simulink model "euler321_I2B_12B_with_contracts_ALL_PP"  (R2017b)
settings: Solver=FixedStepDiscrete  StartTime=0.0  StopTime=10.0  FixedStep=0.010000  RelTol=1e-3  EnableMultiTasking=on
model workspace (MAT data in the model file):
  ContractValidatorBlocksMap = containers.Map
  ContractValidatorBlocksMap.serialization.keys = {'euler321_I2B_12B_with_contracts/euler321_I2B_12B_euler321_Spec/validator', 'euler321_I2B_12B_with_contracts_ALL/euler321_I2B_12B_euler321_Spec/validator'}
  ContractValidatorBlocksMap.serialization.values{1}.block = 'euler321_I2B_12B_with_contracts/euler321_I2B_12B_euler321_Spec/validator'
  ContractValidatorBlocksMap.serialization.values{1}.assumePorts = 0
  ContractValidatorBlocksMap.serialization.values{1}.guaranteePorts = 20
  ContractValidatorBlocksMap.serialization.values{1}.modeBlocksPorts = 0
  ContractValidatorBlocksMap.serialization.values{1}.portHandles.Inport = [576.090576172 577.090576172 578.090576172 579.090576172 580.090576172 581.090576172 582.090576172 583.090576172 584.090576172 585.090576172 586.090576172 587.090576172 588.090576172 589.090576172 590.090576172 591.090576172 592.090576172 593.090576172 594.090576172 595.090576172]
  ContractValidatorBlocksMap.serialization.values{1}.portHandles.Outport = 596.090576172
  ContractValidatorBlocksMap.serialization.values{1}.portHandles.Enable = []
  ContractValidatorBlocksMap.serialization.values{1}.portHandles.Trigger = []
  ContractValidatorBlocksMap.serialization.values{1}.portHandles.State = []
  ContractValidatorBlocksMap.serialization.values{1}.portHandles.LConn = []
  ContractValidatorBlocksMap.serialization.values{1}.portHandles.RConn = []
  ContractValidatorBlocksMap.serialization.values{1}.portHandles.Ifaction = []
  ContractValidatorBlocksMap.serialization.values{1}.portHandles.Reset = []
  ContractValidatorBlocksMap.serialization.values{1}.portConnectivity(1).Type = '1'
  ContractValidatorBlocksMap.serialization.values{1}.portConnectivity(1).Position = [6680 -1090]
  ContractValidatorBlocksMap.serialization.values{1}.portConnectivity(1).SrcBlock = 1677.00183105
  ContractValidatorBlocksMap.serialization.values{1}.portConnectivity(1).SrcPort = 0
  ContractValidatorBlocksMap.serialization.values{1}.portConnectivity(1).DstBlock = []
  ContractValidatorBlocksMap.serialization.values{1}.portConnectivity(1).DstPort = []
  ContractValidatorBlocksMap.serialization.values{1}.portConnectivity(2).Type = '2'
  ContractValidatorBlocksMap.serialization.values{1}.portConnectivity(2).Position = [6680 -1025]
  ContractValidatorBlocksMap.serialization.values{1}.portConnectivity(2).SrcBlock = 1681.00183105
  ContractValidatorBlocksMap.serialization.values{1}.portConnectivity(2).SrcPort = 0
  ContractValidatorBlocksMap.serialization.values{1}.portConnectivity(2).DstBlock = []
  ContractValidatorBlocksMap.serialization.values{1}.portConnectivity(2).DstPort = []
  ContractValidatorBlocksMap.serialization.values{1}.portConnectivity(3).Type = '3'
  ContractValidatorBlocksMap.serialization.values{1}.portConnectivity(3).Position = [6680 -960]
  ContractValidatorBlocksMap.serialization.values{1}.portConnectivity(3).SrcBlock = 1685.00170898
  ContractValidatorBlocksMap.serialization.values{1}.portConnectivity(3).SrcPort = 0
  ContractValidatorBlocksMap.serialization.values{1}.portConnectivity(3).DstBlock = []
  ContractValidatorBlocksMap.serialization.values{1}.portConnectivity(3).DstPort = []
  ContractValidatorBlocksMap.serialization.values{1}.portConnectivity(4).Type = '4'
  ContractValidatorBlocksMap.serialization.values{1}.portConnectivity(4).Position = [6680 -895]
  ContractValidatorBlocksMap.serialization.values{1}.portConnectivity(4).SrcBlock = 1689.00183105
  ContractValidatorBlocksMap.serialization.values{1}.portConnectivity(4).SrcPort = 0
  ContractValidatorBlocksMap.serialization.values{1}.portConnectivity(4).DstBlock = []
  ContractValidatorBlocksMap.serialization.values{1}.portConnectivity(4).DstPort = []
  ContractValidatorBlocksMap.serialization.values{1}.portConnectivity(5).Type = '5'
  ContractValidatorBlocksMap.serialization.values{1}.portConnectivity(5).Position = [6680 -830]
  ContractValidatorBlocksMap.serialization.values{1}.portConnectivity(5).SrcBlock = 1693.00146484
  ContractValidatorBlocksMap.serialization.values{1}.portConnectivity(5).SrcPort = 0
  ContractValidatorBlocksMap.serialization.values{1}.portConnectivity(5).DstBlock = []
  ContractValidatorBlocksMap.serialization.values{1}.portConnectivity(5).DstPort = []
  ContractValidatorBlocksMap.serialization.values{1}.portConnectivity(6).Type = '6'
  ContractValidatorBlocksMap.serialization.values{1}.portConnectivity(6).Position = [6680 -765]
  ContractValidatorBlocksMap.serialization.values{1}.portConnectivity(6).SrcBlock = 1697.00146484
  ContractValidatorBlocksMap.serialization.values{1}.portConnectivity(6).SrcPort = 0
  ContractValidatorBlocksMap.serialization.values{1}.portConnectivity(6).DstBlock = []
  ContractValidatorBlocksMap.serialization.values{1}.portConnectivity(6).DstPort = []
  ContractValidatorBlocksMap.serialization.values{1}.portConnectivity(7).Type = '7'
  ContractValidatorBlocksMap.serialization.values{1}.portConnectivity(7).Position = [6680 -700]
  ContractValidatorBlocksMap.serialization.values{1}.portConnectivity(7).SrcBlock = 1701.00183105
  ContractValidatorBlocksMap.serialization.values{1}.portConnectivity(7).SrcPort = 0
  ContractValidatorBlocksMap.serialization.values{1}.portConnectivity(7).DstBlock = []
  ContractValidatorBlocksMap.serialization.values{1}.portConnectivity(7).DstPort = []
  ContractValidatorBlocksMap.serialization.values{1}.portConnectivity(8).Type = '8'
  ContractValidatorBlocksMap.serialization.values{1}.portConnectivity(8).Position = [6680 -635]
  ContractValidatorBlocksMap.serialization.values{1}.portConnectivity(8).SrcBlock = 1705.00183105
  ContractValidatorBlocksMap.serialization.values{1}.portConnectivity(8).SrcPort = 0
  ContractValidatorBlocksMap.serialization.values{1}.portConnectivity(8).DstBlock = []
  ContractValidatorBlocksMap.serialization.values{1}.portConnectivity(8).DstPort = []
  ContractValidatorBlocksMap.serialization.values{1}.portConnectivity(9).Type = '9'
  ContractValidatorBlocksMap.serialization.values{1}.portConnectivity(9).Position = [6680 -570]
  ContractValidatorBlocksMap.serialization.values{1}.portConnectivity(9).SrcBlock = 1709.00134277
  ContractValidatorBlocksMap.serialization.values{1}.portConnectivity(9).SrcPort = 0
  ContractValidatorBlocksMap.serialization.values{1}.portConnectivity(9).DstBlock = []
  ContractValidatorBlocksMap.serialization.values{1}.portConnectivity(9).DstPort = []
  ContractValidatorBlocksMap.serialization.values{1}.portConnectivity(10).Type = '10'
  ContractValidatorBlocksMap.serialization.values{1}.portConnectivity(10).Position = [6680 -505]
  ContractValidatorBlocksMap.serialization.values{1}.portConnectivity(10).SrcBlock = 1713.00170898
  ContractValidatorBlocksMap.serialization.values{1}.portConnectivity(10).SrcPort = 0
  ContractValidatorBlocksMap.serialization.values{1}.portConnectivity(10).DstBlock = []
  ContractValidatorBlocksMap.serialization.values{1}.portConnectivity(10).DstPort = []
  ContractValidatorBlocksMap.serialization.values{1}.portConnectivity(11).Type = '11'
  ContractValidatorBlocksMap.serialization.values{1}.portConnectivity(11).Position = [6680 -440]
  ContractValidatorBlocksMap.serialization.values{1}.portConnectivity(11).SrcBlock = 1717.00183105
  ContractValidatorBlocksMap.serialization.values{1}.portConnectivity(11).SrcPort = 0
  ContractValidatorBlocksMap.serialization.values{1}.portConnectivity(11).DstBlock = []
  ContractValidatorBlocksMap.serialization.values{1}.portConnectivity(11).DstPort = []
  ContractValidatorBlocksMap.serialization.values{1}.portConnectivity(12).Type = '12'
  ContractValidatorBlocksMap.serialization.values{1}.portConnectivity(12).Position = [6680 -375]
  ContractValidatorBlocksMap.serialization.values{1}.portConnectivity(12).SrcBlock = 1721.00146484
  ContractValidatorBlocksMap.serialization.values{1}.portConnectivity(12).SrcPort = 0
  ContractValidatorBlocksMap.serialization.values{1}.portConnectivity(12).DstBlock = []
  ContractValidatorBlocksMap.serialization.values{1}.portConnectivity(12).DstPort = []
  ContractValidatorBlocksMap.serialization.values{1}.portConnectivity(13).Type = '13'
  ContractValidatorBlocksMap.serialization.values{1}.portConnectivity(13).Position = [6680 -310]
  ContractValidatorBlocksMap.serialization.values{1}.portConnectivity(13).SrcBlock = 1725.00170898
  ContractValidatorBlocksMap.serialization.values{1}.portConnectivity(13).SrcPort = 0
  ContractValidatorBlocksMap.serialization.values{1}.portConnectivity(13).DstBlock = []
  ContractValidatorBlocksMap.serialization.values{1}.portConnectivity(13).DstPort = []
  ContractValidatorBlocksMap.serialization.values{1}.portConnectivity(14).Type = '14'
  ContractValidatorBlocksMap.serialization.values{1}.portConnectivity(14).Position = [6680 -245]
  ContractValidatorBlocksMap.serialization.values{1}.portConnectivity(14).SrcBlock = 1729.00146484
  ContractValidatorBlocksMap.serialization.values{1}.portConnectivity(14).SrcPort = 0
  ContractValidatorBlocksMap.serialization.values{1}.portConnectivity(14).DstBlock = []
  ContractValidatorBlocksMap.serialization.values{1}.portConnectivity(14).DstPort = []
  ContractValidatorBlocksMap.serialization.values{1}.portConnectivity(15).Type = '15'
  ContractValidatorBlocksMap.serialization.values{1}.portConnectivity(15).Position = [6680 -180]
  ContractValidatorBlocksMap.serialization.values{1}.portConnectivity(15).SrcBlock = 1733.00183105
  ContractValidatorBlocksMap.serialization.values{1}.portConnectivity(15).SrcPort = 0
  ContractValidatorBlocksMap.serialization.values{1}.portConnectivity(15).DstBlock = []
  ContractValidatorBlocksMap.serialization.values{1}.portConnectivity(15).DstPort = []
  ContractValidatorBlocksMap.serialization.values{1}.portConnectivity(16).Type = '16'
  ContractValidatorBlocksMap.serialization.values{1}.portConnectivity(16).Position = [6680 -115]
  ContractValidatorBlocksMap.serialization.values{1}.portConnectivity(16).SrcBlock = 1737.00134277
  ContractValidatorBlocksMap.serialization.values{1}.portConnectivity(16).SrcPort = 0
  ContractValidatorBlocksMap.serialization.values{1}.portConnectivity(16).DstBlock = []
  ContractValidatorBlocksMap.serialization.values{1}.portConnectivity(16).DstPort = []
  ContractValidatorBlocksMap.serialization.values{1}.portConnectivity(17).Type = '17'
  ContractValidatorBlocksMap.serialization.values{1}.portConnectivity(17).Position = [6680 -50]
  ContractValidatorBlocksMap.serialization.values{1}.portConnectivity(17).SrcBlock = 1741.00146484
  ContractValidatorBlocksMap.serialization.values{1}.portConnectivity(17).SrcPort = 0
  ContractValidatorBlocksMap.serialization.values{1}.portConnectivity(17).DstBlock = []
  ContractValidatorBlocksMap.serialization.values{1}.portConnectivity(17).DstPort = []
  ContractValidatorBlocksMap.serialization.values{1}.portConnectivity(18).Type = '18'
  ContractValidatorBlocksMap.serialization.values{1}.portConnectivity(18).Position = [6680 15]
  ContractValidatorBlocksMap.serialization.values{1}.portConnectivity(18).SrcBlock = 1745.00183105
  ContractValidatorBlocksMap.serialization.values{1}.portConnectivity(18).SrcPort = 0
  ContractValidatorBlocksMap.serialization.values{1}.portConnectivity(18).DstBlock = []
  ContractValidatorBlocksMap.serialization.values{1}.portConnectivity(18).DstPort = []
  ContractValidatorBlocksMap.serialization.values{1}.portConnectivity(19).Type = '19'
  ContractValidatorBlocksMap.serialization.values{1}.portConnectivity(19).Position = [6680 80]
  ContractValidatorBlocksMap.serialization.values{1}.portConnectivity(19).SrcBlock = 1834.0020752
  ContractValidatorBlocksMap.serialization.values{1}.portConnectivity(19).SrcPort = 0
  ContractValidatorBlocksMap.serialization.values{1}.portConnectivity(19).DstBlock = []
  ContractValidatorBlocksMap.serialization.values{1}.portConnectivity(19).DstPort = []
  ContractValidatorBlocksMap.serialization.values{1}.portConnectivity(20).Type = '20'
  ContractValidatorBlocksMap.serialization.values{1}.portConnectivity(20).Position = [6680 145]
  ContractValidatorBlocksMap.serialization.values{1}.portConnectivity(20).SrcBlock = 1838.00195312
  ContractValidatorBlocksMap.serialization.values{1}.portConnectivity(20).SrcPort = 0
  ContractValidatorBlocksMap.serialization.values{1}.portConnectivity(20).DstBlock = []
  ContractValidatorBlocksMap.serialization.values{1}.portConnectivity(20).DstPort = []
  ContractValidatorBlocksMap.serialization.values{1}.portConnectivity(21).Type = '1'
  ContractValidatorBlocksMap.serialization.values{1}.portConnectivity(21).Position = [6855 -470]
  ContractValidatorBlocksMap.serialization.values{1}.portConnectivity(21).SrcBlock = []
  ContractValidatorBlocksMap.serialization.values{1}.portConnectivity(21).SrcPort = []
  ContractValidatorBlocksMap.serialization.values{1}.portConnectivity(21).DstBlock = 2655.00268555
  ContractValidatorBlocksMap.serialization.values{1}.portConnectivity(21).DstPort = 0
  ContractValidatorBlocksMap.serialization.values{2}.block = 'euler321_I2B_12B_with_contracts_ALL/euler321_I2B_12B_euler321_Spec/validator'
  ContractValidatorBlocksMap.serialization.values{2}.assumePorts = 0
  ContractValidatorBlocksMap.serialization.values{2}.guaranteePorts = 20
  ContractValidatorBlocksMap.serialization.values{2}.modeBlocksPorts = 0
  ContractValidatorBlocksMap.serialization.values{2}.portHandles.Inport = [10350.0007324 10351.0007324 10352.0007324 10353.0007324 10354.0007324 10355.0007324 10356.0007324 10357.0007324 10358.0007324 10359.0007324 10360.0007324 10361.0007324 10362.0007324 10363.0007324 10364.0007324 10365.0007324 10366.0007324 10367.0007324 10368.0007324 10369.0007324]
  ContractValidatorBlocksMap.serialization.values{2}.portHandles.Outport = 10370.0007324
  ContractValidatorBlocksMap.serialization.values{2}.portHandles.Enable = []
  ContractValidatorBlocksMap.serialization.values{2}.portHandles.Trigger = []
  ContractValidatorBlocksMap.serialization.values{2}.portHandles.State = []
  ContractValidatorBlocksMap.serialization.values{2}.portHandles.LConn = []
  ContractValidatorBlocksMap.serialization.values{2}.portHandles.RConn = []
  ContractValidatorBlocksMap.serialization.values{2}.portHandles.Ifaction = []
  ContractValidatorBlocksMap.serialization.values{2}.portHandles.Reset = []
  ContractValidatorBlocksMap.serialization.values{2}.portConnectivity(1).Type = '1'
  ContractValidatorBlocksMap.serialization.values{2}.portConnectivity(1).Position = [6680 -1090]
  ContractValidatorBlocksMap.serialization.values{2}.portConnectivity(1).SrcBlock = 9376.00109863
  ContractValidatorBlocksMap.serialization.values{2}.portConnectivity(1).SrcPort = 0
  ContractValidatorBlocksMap.serialization.values{2}.portConnectivity(1).DstBlock = []
  ContractValidatorBlocksMap.serialization.values{2}.portConnectivity(1).DstPort = []
  ContractValidatorBlocksMap.serialization.values{2}.portConnectivity(2).Type = '2'
  ContractValidatorBlocksMap.serialization.values{2}.portConnectivity(2).Position = [6680 -1025]
  ContractValidatorBlocksMap.serialization.values{2}.portConnectivity(2).SrcBlock = 9380.00109863
  ContractValidatorBlocksMap.serialization.values{2}.portConnectivity(2).SrcPort = 0
  ContractValidatorBlocksMap.serialization.values{2}.portConnectivity(2).DstBlock = []
  ContractValidatorBlocksMap.serialization.values{2}.portConnectivity(2).DstPort = []
  ContractValidatorBlocksMap.serialization.values{2}.portConnectivity(3).Type = '3'
  ContractValidatorBlocksMap.serialization.values{2}.portConnectivity(3).Position = [6680 -960]
  ContractValidatorBlocksMap.serialization.values{2}.portConnectivity(3).SrcBlock = 9384.00109863
  ContractValidatorBlocksMap.serialization.values{2}.portConnectivity(3).SrcPort = 0
  ContractValidatorBlocksMap.serialization.values{2}.portConnectivity(3).DstBlock = []
  ContractValidatorBlocksMap.serialization.values{2}.portConnectivity(3).DstPort = []
  ContractValidatorBlocksMap.serialization.values{2}.portConnectivity(4).Type = '4'
  ContractValidatorBlocksMap.serialization.values{2}.portConnectivity(4).Position = [6680 -895]
  ContractValidatorBlocksMap.serialization.values{2}.portConnectivity(4).SrcBlock = 9388.00109863
  ContractValidatorBlocksMap.serialization.values{2}.portConnectivity(4).SrcPort = 0
  ContractValidatorBlocksMap.serialization.values{2}.portConnectivity(4).DstBlock = []
  ContractValidatorBlocksMap.serialization.values{2}.portConnectivity(4).DstPort = []
  ContractValidatorBlocksMap.serialization.values{2}.portConnectivity(5).Type = '5'
  ContractValidatorBlocksMap.serialization.values{2}.portConnectivity(5).Position = [6680 -830]
  ContractValidatorBlocksMap.serialization.values{2}.portConnectivity(5).SrcBlock = 9392.00109863
  ContractValidatorBlocksMap.serialization.values{2}.portConnectivity(5).SrcPort = 0
  ContractValidatorBlocksMap.serialization.values{2}.portConnectivity(5).DstBlock = []
  ContractValidatorBlocksMap.serialization.values{2}.portConnectivity(5).DstPort = []
  ContractValidatorBlocksMap.serialization.values{2}.portConnectivity(6).Type = '6'
  ContractValidatorBlocksMap.serialization.values{2}.portConnectivity(6).Position = [6680 -765]
  ContractValidatorBlocksMap.serialization.values{2}.portConnectivity(6).SrcBlock = 9396.00109863
  ContractValidatorBlocksMap.serialization.values{2}.portConnectivity(6).SrcPort = 0
  ContractValidatorBlocksMap.serialization.values{2}.portConnectivity(6).DstBlock = []
  ContractValidatorBlocksMap.serialization.values{2}.portConnectivity(6).DstPort = []
  ContractValidatorBlocksMap.serialization.values{2}.portConnectivity(7).Type = '7'
  ContractValidatorBlocksMap.serialization.values{2}.portConnectivity(7).Position = [6680 -700]
  ContractValidatorBlocksMap.serialization.values{2}.portConnectivity(7).SrcBlock = 9400.00109863
  ContractValidatorBlocksMap.serialization.values{2}.portConnectivity(7).SrcPort = 0
  ContractValidatorBlocksMap.serialization.values{2}.portConnectivity(7).DstBlock = []
  ContractValidatorBlocksMap.serialization.values{2}.portConnectivity(7).DstPort = []
  ContractValidatorBlocksMap.serialization.values{2}.portConnectivity(8).Type = '8'
  ContractValidatorBlocksMap.serialization.values{2}.portConnectivity(8).Position = [6680 -635]
  ContractValidatorBlocksMap.serialization.values{2}.portConnectivity(8).SrcBlock = 9404.00109863
  ContractValidatorBlocksMap.serialization.values{2}.portConnectivity(8).SrcPort = 0
  ContractValidatorBlocksMap.serialization.values{2}.portConnectivity(8).DstBlock = []
  ContractValidatorBlocksMap.serialization.values{2}.portConnectivity(8).DstPort = []
  ContractValidatorBlocksMap.serialization.values{2}.portConnectivity(9).Type = '9'
  ContractValidatorBlocksMap.serialization.values{2}.portConnectivity(9).Position = [6680 -570]
  ContractValidatorBlocksMap.serialization.values{2}.portConnectivity(9).SrcBlock = 9408.00109863
  ContractValidatorBlocksMap.serialization.values{2}.portConnectivity(9).SrcPort = 0
  ContractValidatorBlocksMap.serialization.values{2}.portConnectivity(9).DstBlock = []
  ContractValidatorBlocksMap.serialization.values{2}.portConnectivity(9).DstPort = []
  ContractValidatorBlocksMap.serialization.values{2}.portConnectivity(10).Type = '10'
  ContractValidatorBlocksMap.serialization.values{2}.portConnectivity(10).Position = [6680 -505]
  ContractValidatorBlocksMap.serialization.values{2}.portConnectivity(10).SrcBlock = 9412.00109863
  ContractValidatorBlocksMap.serialization.values{2}.portConnectivity(10).SrcPort = 0
  ContractValidatorBlocksMap.serialization.values{2}.portConnectivity(10).DstBlock = []
  ContractValidatorBlocksMap.serialization.values{2}.portConnectivity(10).DstPort = []
  ContractValidatorBlocksMap.serialization.values{2}.portConnectivity(11).Type = '11'
  ContractValidatorBlocksMap.serialization.values{2}.portConnectivity(11).Position = [6680 -440]
  ContractValidatorBlocksMap.serialization.values{2}.portConnectivity(11).SrcBlock = 9416.00109863
  ContractValidatorBlocksMap.serialization.values{2}.portConnectivity(11).SrcPort = 0
  ContractValidatorBlocksMap.serialization.values{2}.portConnectivity(11).DstBlock = []
  ContractValidatorBlocksMap.serialization.values{2}.portConnectivity(11).DstPort = []
  ContractValidatorBlocksMap.serialization.values{2}.portConnectivity(12).Type = '12'
  ContractValidatorBlocksMap.serialization.values{2}.portConnectivity(12).Position = [6680 -375]
  ContractValidatorBlocksMap.serialization.values{2}.portConnectivity(12).SrcBlock = 9420.00109863
  ContractValidatorBlocksMap.serialization.values{2}.portConnectivity(12).SrcPort = 0
  ContractValidatorBlocksMap.serialization.values{2}.portConnectivity(12).DstBlock = []
  ContractValidatorBlocksMap.serialization.values{2}.portConnectivity(12).DstPort = []
  ContractValidatorBlocksMap.serialization.values{2}.portConnectivity(13).Type = '13'
  ContractValidatorBlocksMap.serialization.values{2}.portConnectivity(13).Position = [6680 -310]
  ContractValidatorBlocksMap.serialization.values{2}.portConnectivity(13).SrcBlock = 9424.00109863
  ContractValidatorBlocksMap.serialization.values{2}.portConnectivity(13).SrcPort = 0
  ContractValidatorBlocksMap.serialization.values{2}.portConnectivity(13).DstBlock = []
  ContractValidatorBlocksMap.serialization.values{2}.portConnectivity(13).DstPort = []
  ContractValidatorBlocksMap.serialization.values{2}.portConnectivity(14).Type = '14'
  ContractValidatorBlocksMap.serialization.values{2}.portConnectivity(14).Position = [6680 -245]
  ContractValidatorBlocksMap.serialization.values{2}.portConnectivity(14).SrcBlock = 9428.00109863
  ContractValidatorBlocksMap.serialization.values{2}.portConnectivity(14).SrcPort = 0
  ContractValidatorBlocksMap.serialization.values{2}.portConnectivity(14).DstBlock = []
  ContractValidatorBlocksMap.serialization.values{2}.portConnectivity(14).DstPort = []
  ContractValidatorBlocksMap.serialization.values{2}.portConnectivity(15).Type = '15'
  ContractValidatorBlocksMap.serialization.values{2}.portConnectivity(15).Position = [6680 -180]
  ContractValidatorBlocksMap.serialization.values{2}.portConnectivity(15).SrcBlock = 9432.00109863
  ContractValidatorBlocksMap.serialization.values{2}.portConnectivity(15).SrcPort = 0
  ContractValidatorBlocksMap.serialization.values{2}.portConnectivity(15).DstBlock = []
  ContractValidatorBlocksMap.serialization.values{2}.portConnectivity(15).DstPort = []
  ContractValidatorBlocksMap.serialization.values{2}.portConnectivity(16).Type = '16'
  ContractValidatorBlocksMap.serialization.values{2}.portConnectivity(16).Position = [6680 -115]
  ContractValidatorBlocksMap.serialization.values{2}.portConnectivity(16).SrcBlock = 9436.00109863
  ContractValidatorBlocksMap.serialization.values{2}.portConnectivity(16).SrcPort = 0
  ContractValidatorBlocksMap.serialization.values{2}.portConnectivity(16).DstBlock = []
  ContractValidatorBlocksMap.serialization.values{2}.portConnectivity(16).DstPort = []
  ContractValidatorBlocksMap.serialization.values{2}.portConnectivity(17).Type = '17'
  ContractValidatorBlocksMap.serialization.values{2}.portConnectivity(17).Position = [6680 -50]
  ContractValidatorBlocksMap.serialization.values{2}.portConnectivity(17).SrcBlock = 9440.00109863
  ContractValidatorBlocksMap.serialization.values{2}.portConnectivity(17).SrcPort = 0
  ContractValidatorBlocksMap.serialization.values{2}.portConnectivity(17).DstBlock = []
  ContractValidatorBlocksMap.serialization.values{2}.portConnectivity(17).DstPort = []
  ContractValidatorBlocksMap.serialization.values{2}.portConnectivity(18).Type = '18'
  ContractValidatorBlocksMap.serialization.values{2}.portConnectivity(18).Position = [6680 15]
  ContractValidatorBlocksMap.serialization.values{2}.portConnectivity(18).SrcBlock = 9444.00109863
  ContractValidatorBlocksMap.serialization.values{2}.portConnectivity(18).SrcPort = 0
  ContractValidatorBlocksMap.serialization.values{2}.portConnectivity(18).DstBlock = []
  ContractValidatorBlocksMap.serialization.values{2}.portConnectivity(18).DstPort = []
  ContractValidatorBlocksMap.serialization.values{2}.portConnectivity(19).Type = '19'
  ContractValidatorBlocksMap.serialization.values{2}.portConnectivity(19).Position = [6680 80]
  ContractValidatorBlocksMap.serialization.values{2}.portConnectivity(19).SrcBlock = 9448.00109863
  ContractValidatorBlocksMap.serialization.values{2}.portConnectivity(19).SrcPort = 0
  ContractValidatorBlocksMap.serialization.values{2}.portConnectivity(19).DstBlock = []
  ContractValidatorBlocksMap.serialization.values{2}.portConnectivity(19).DstPort = []
  ContractValidatorBlocksMap.serialization.values{2}.portConnectivity(20).Type = '20'
  ContractValidatorBlocksMap.serialization.values{2}.portConnectivity(20).Position = [6680 145]
  ContractValidatorBlocksMap.serialization.values{2}.portConnectivity(20).SrcBlock = 9452.00109863
  ContractValidatorBlocksMap.serialization.values{2}.portConnectivity(20).SrcPort = 0
  ContractValidatorBlocksMap.serialization.values{2}.portConnectivity(20).DstBlock = []
  ContractValidatorBlocksMap.serialization.values{2}.portConnectivity(20).DstPort = []
  ContractValidatorBlocksMap.serialization.values{2}.portConnectivity(21).Type = '1'
  ContractValidatorBlocksMap.serialization.values{2}.portConnectivity(21).Position = [6855 -470]
  ContractValidatorBlocksMap.serialization.values{2}.portConnectivity(21).SrcBlock = []
  ContractValidatorBlocksMap.serialization.values{2}.portConnectivity(21).SrcPort = []
  ContractValidatorBlocksMap.serialization.values{2}.portConnectivity(21).DstBlock = 9756.01013184
  ContractValidatorBlocksMap.serialization.values{2}.portConnectivity(21).DstPort = 0
  ContractValidatorBlocksMap.serialization.uniformity = 0
  ContractValidatorBlocksMap.serialization.keyType = 'char'
  ContractValidatorBlocksMap.serialization.valueType = 'any'
  already_pp = 1
undefined symbols (not defined in the file): contractAfterSimulation, contractBeforeSimulation, ContractBlock, ContractGuaranteeBlock, ContractValidatorBlock, saveValidatorParameters
(part 1 of 2)
settings Model: Creator=elliocm  LastModifiedBy=hbourbou
settings DataIOCC: LimitDataPoints=on  SaveFormat=StructureWithTime  SignalLoggingSaveFormat=ModelDataLogs
settings OptimizationCC: ExpressionDepthLimit=2147483647  LifeSpan=inf
settings DebuggingCC: AlgebraicLoopMsg=error  ArtificialAlgebraicLoopMsg=error  UnderspecifiedInitializationDetection=Classic  MergeDetectMultiDrivingBlocksExec=none  SolverPrmCheckMsg=warning  SingleTaskRateTransMsg=error  FcnCallInpInsideContextMsg=warning  StateNameClashWarn=warning  SFUnexpectedBacktrackingDiag=warning  SFNoUnconditionalDefaultTransitionDiag=warning  SFExecutionAtInitializationDiag=none
settings HardwareCC: ProdBitPerPointer=32  ProdBitPerSizeT=32  ProdBitPerPtrDiffT=32  ProdLargestAtomicFloat=None  ProdIntDivRoundTo=Undefined  ProdEndianess=Unspecified  ProdWordSize=32  ProdHWDeviceType=32-bit Generic
settings ModelReferenceCC: PropagateSignalLabelsOutOfModel=off
settings CodeAppCC: StateflowObjectComments=on
settings GRTTargetCC: TargetLangStandard=C89/C90 (ANSI)  GeneratePreprocessorConditionals=Disable all  CombineOutputUpdateFcns=off  GRTInterface=on
settings ConfigComp: CovMetricSettings=dw  CovHtmlReporting=on  CovSaveCumulativeToWorkspaceVar=on  CovSaveSingleToWorkspaceVar=on  CovExternalEMLEnable=off

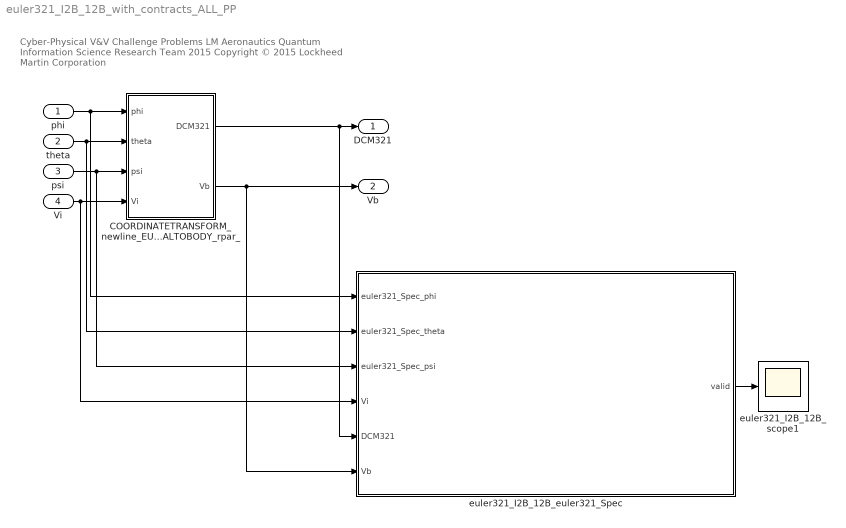
== system euler321_I2B_12B_with_contracts_ALL_PP ==
  note: Cyber-Physical V&V Challenge Problems
      | LM Aeronautics Quantum Information Science Research Team 2015
      | Copyright © 2015 Lockheed Martin Corporation
  phi : Inport  OutDataTypeStr=double
  theta : Inport  Port=2  OutDataTypeStr=double
  psi : Inport  Port=3  OutDataTypeStr=double
  Vi : Inport  Port=4  OutDataTypeStr=double  PortDimensions=3
  COORDINATETRANSFORM_newline_EULER321_newline__lpar_INERTIALTOBODY_rpar_ : Subsystem  TreatAsAtomicUnit=on
  euler321_I2B_12B_euler321_Spec : Subsystem  TreatAsAtomicUnit=on  mask(ContractBlock){ContractBlockType=ContractBlock}
      mask init:
      | set_param(gcb, 'LinkStatus', 'none');
      mask DialogControl DescTextVar Prompt: Contract block
      mask Display:
      | text(0.5, 0.5, '{\bf\fontsize{20}Contract}', 'hor', 'center', 'texmode','on');
      | blocks = find_system(gcb, 'LookUnderMasks','all', 'SearchDepth',1,'BlockType','Inport');
      | for i = 1 : length(blocks)
      |     blockName = get_param(blocks(i), 'Name');
      |     [path, blockName] = fileparts(char(blockName));
      |     port_label('input', i, blockName);
      | end
      | 
      | blocks = find_system(gcb, 'LookUnderMasks','all', 'SearchDepth',1,'BlockType','Outport');
      | for i = 1 : length(blocks)
      |     blockName = get_param(blocks(i), 'Name');
      |     [path, blockName] = fileparts(char(blockName));
      |     port_label('output', i, blockName);
      | end
  euler321_I2B_12B_scope1 : Scope
  DCM321 : Outport  VectorParamsAs1DForOutWhenUnconnected=off
  Vb : Outport  Port=2  VectorParamsAs1DForOutWhenUnconnected=off
  wires:
  COORDINATETRANSFORM_newline_EULER321_newline__lpar_INERTIALTOBODY_rpar_/1(DCM321) -> euler321_I2B_12B_euler321_Spec/5(DCM321), DCM321/1
  COORDINATETRANSFORM_newline_EULER321_newline__lpar_INERTIALTOBODY_rpar_/2(Vb) -> euler321_I2B_12B_euler321_Spec/6(Vb), Vb/1
  phi/1 -> euler321_I2B_12B_euler321_Spec/1(euler321_Spec_phi), COORDINATETRANSFORM_newline_EULER321_newline__lpar_INERTIALTOBODY_rpar_/1(phi)
  theta/1 -> euler321_I2B_12B_euler321_Spec/2(euler321_Spec_theta), COORDINATETRANSFORM_newline_EULER321_newline__lpar_INERTIALTOBODY_rpar_/2(theta)
  psi/1 -> euler321_I2B_12B_euler321_Spec/3(euler321_Spec_psi), COORDINATETRANSFORM_newline_EULER321_newline__lpar_INERTIALTOBODY_rpar_/3(psi)
  Vi/1 -> COORDINATETRANSFORM_newline_EULER321_newline__lpar_INERTIALTOBODY_rpar_/4(Vi), euler321_I2B_12B_euler321_Spec/4(Vi)
  euler321_I2B_12B_euler321_Spec/1(valid) -> euler321_I2B_12B_scope1/1

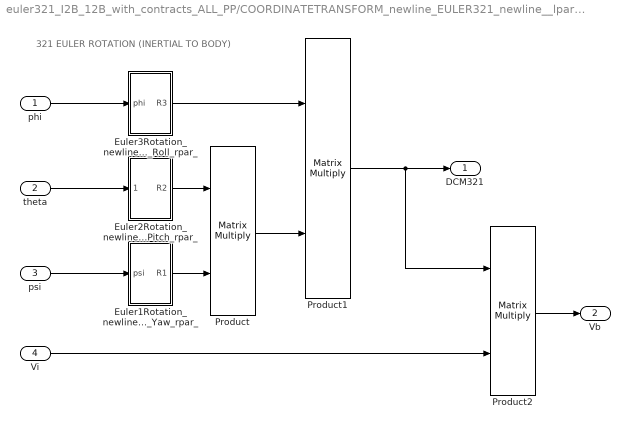
== system euler321_I2B_12B_with_contracts_ALL_PP/COORDINATETRANSFORM_newline_EULER321_newline__lpar_INERTIALTOBODY_rpar_ ==
  note: 321 EULER ROTATION (INERTIAL TO BODY)
  phi : Inport
  theta : Inport  Port=2
  psi : Inport  Port=3
  Vi : Inport  Port=4
  Euler1Rotation_newline__lpar_Yaw_rpar_ : Subsystem  TreatAsAtomicUnit=on
  Euler2Rotation_newline__lpar_Pitch_rpar_ : Subsystem  TreatAsAtomicUnit=on
  Euler3Rotation_newline__lpar_Roll_rpar_ : Subsystem  TreatAsAtomicUnit=on
  Product : Product  Multiplication=Matrix(*)  RndMeth=Zero
  Product1 : Product  Multiplication=Matrix(*)  RndMeth=Zero
  Product2 : Product  Multiplication=Matrix(*)  RndMeth=Zero
  DCM321 : Outport  VectorParamsAs1DForOutWhenUnconnected=off
  Vb : Outport  Port=2  VectorParamsAs1DForOutWhenUnconnected=off
  wires:
  Euler2Rotation_newline__lpar_Pitch_rpar_/1(R2) -> Product/1
  Euler1Rotation_newline__lpar_Yaw_rpar_/1(R1) -> Product/2
  Euler3Rotation_newline__lpar_Roll_rpar_/1(R3) -> Product1/1
  Product/1 -> Product1/2
  Product1/1 -> DCM321/1, Product2/1
  Product2/1 -> Vb/1
  phi/1 -> Euler3Rotation_newline__lpar_Roll_rpar_/1(phi)
  theta/1 -> Euler2Rotation_newline__lpar_Pitch_rpar_/1(theta)
  psi/1 -> Euler1Rotation_newline__lpar_Yaw_rpar_/1(psi)
  Vi/1 -> Product2/2

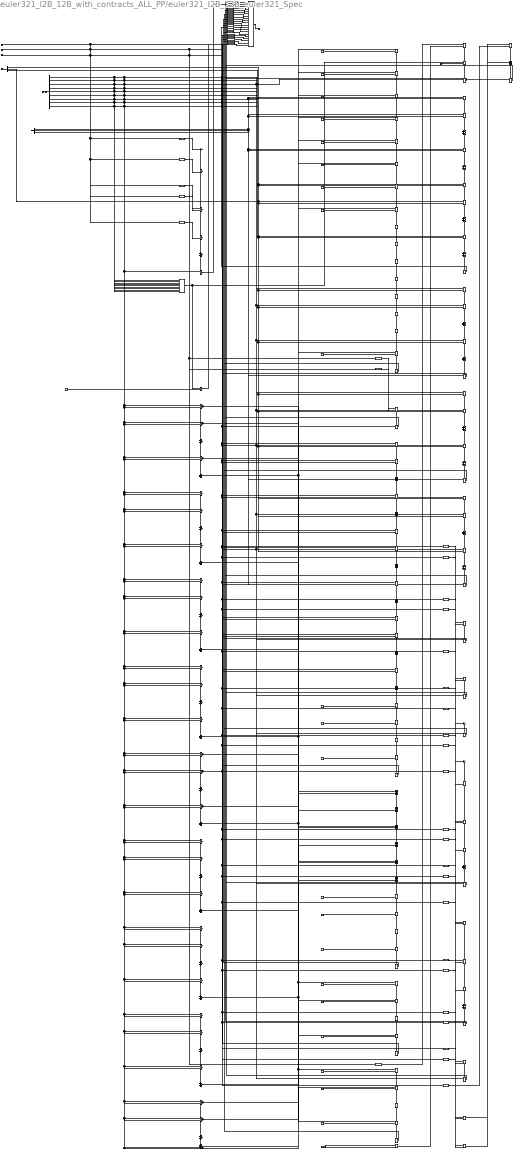
== system euler321_I2B_12B_with_contracts_ALL_PP/euler321_I2B_12B_euler321_Spec ==
  euler321_Spec_phi : Inport  OutDataTypeStr=double
  euler321_Spec_theta : Inport  Port=2  OutDataTypeStr=double
  euler321_Spec_psi : Inport  Port=3  OutDataTypeStr=double
  Vi : Inport  Port=4
  DCM321 : Inport  Port=5
  Vb : Inport  Port=6
  Demux : Demux  Outputs=3
  Demux1 : Demux  Outputs=3
  Demux3 : Demux  Outputs=9
  EUL_001_1 : Subsystem  TreatAsAtomicUnit=on  mask(ContractGuaranteeBlock){ContractBlockType=ContractGuaranteeBlock}
      mask init:
      | set_param(gcb, 'LinkStatus', 'none');
      mask DialogControl DescTextVar Prompt: Guarantee block
  EUL_001_2 : Subsystem  TreatAsAtomicUnit=on  mask(ContractGuaranteeBlock){ContractBlockType=ContractGuaranteeBlock}
      mask init:
      | set_param(gcb, 'LinkStatus', 'none');
      mask DialogControl DescTextVar Prompt: Guarantee block
  EUL_001_3 : Subsystem  TreatAsAtomicUnit=on  mask(ContractGuaranteeBlock){ContractBlockType=ContractGuaranteeBlock}
      mask init:
      | set_param(gcb, 'LinkStatus', 'none');
      mask DialogControl DescTextVar Prompt: Guarantee block
  EUL_001_4 : Subsystem  TreatAsAtomicUnit=on  mask(ContractGuaranteeBlock){ContractBlockType=ContractGuaranteeBlock}
      mask init:
      | set_param(gcb, 'LinkStatus', 'none');
      mask DialogControl DescTextVar Prompt: Guarantee block
  EUL_001_5 : Subsystem  TreatAsAtomicUnit=on  mask(ContractGuaranteeBlock){ContractBlockType=ContractGuaranteeBlock}
      mask init:
      | set_param(gcb, 'LinkStatus', 'none');
      mask DialogControl DescTextVar Prompt: Guarantee block
  EUL_001_6 : Subsystem  TreatAsAtomicUnit=on  mask(ContractGuaranteeBlock){ContractBlockType=ContractGuaranteeBlock}
      mask init:
      | set_param(gcb, 'LinkStatus', 'none');
      mask DialogControl DescTextVar Prompt: Guarantee block
  EUL_001_7 : Subsystem  TreatAsAtomicUnit=on  mask(ContractGuaranteeBlock){ContractBlockType=ContractGuaranteeBlock}
      mask init:
      | set_param(gcb, 'LinkStatus', 'none');
      mask DialogControl DescTextVar Prompt: Guarantee block
  EUL_001_8 : Subsystem  TreatAsAtomicUnit=on  mask(ContractGuaranteeBlock){ContractBlockType=ContractGuaranteeBlock}
      mask init:
      | set_param(gcb, 'LinkStatus', 'none');
      mask DialogControl DescTextVar Prompt: Guarantee block
  EUL_001_9 : Subsystem  TreatAsAtomicUnit=on  mask(ContractGuaranteeBlock){ContractBlockType=ContractGuaranteeBlock}
      mask init:
      | set_param(gcb, 'LinkStatus', 'none');
      mask DialogControl DescTextVar Prompt: Guarantee block
  EUL_002_1 : Subsystem  TreatAsAtomicUnit=on  mask(ContractGuaranteeBlock){ContractBlockType=ContractGuaranteeBlock}
      mask init:
      | set_param(gcb, 'LinkStatus', 'none');
      mask DialogControl DescTextVar Prompt: Guarantee block
  EUL_002_2 : Subsystem  TreatAsAtomicUnit=on  mask(ContractGuaranteeBlock){ContractBlockType=ContractGuaranteeBlock}
      mask init:
      | set_param(gcb, 'LinkStatus', 'none');
      mask DialogControl DescTextVar Prompt: Guarantee block
  EUL_002_3 : Subsystem  TreatAsAtomicUnit=on  mask(ContractGuaranteeBlock){ContractBlockType=ContractGuaranteeBlock}
      mask init:
      | set_param(gcb, 'LinkStatus', 'none');
      mask DialogControl DescTextVar Prompt: Guarantee block
  EUL_003 : Subsystem  TreatAsAtomicUnit=on  mask(ContractGuaranteeBlock){ContractBlockType=ContractGuaranteeBlock}
      mask init:
      | set_param(gcb, 'LinkStatus', 'none');
      mask DialogControl DescTextVar Prompt: Guarantee block
  EUL_004 : Subsystem  TreatAsAtomicUnit=on  mask(ContractGuaranteeBlock){ContractBlockType=ContractGuaranteeBlock}
      mask init:
      | set_param(gcb, 'LinkStatus', 'none');
      mask DialogControl DescTextVar Prompt: Guarantee block
  EUL_006_1 : Subsystem  TreatAsAtomicUnit=on  mask(ContractGuaranteeBlock){ContractBlockType=ContractGuaranteeBlock}
      mask init:
      | set_param(gcb, 'LinkStatus', 'none');
      mask DialogControl DescTextVar Prompt: Guarantee block
  EUL_006_2 : Subsystem  TreatAsAtomicUnit=on  mask(ContractGuaranteeBlock){ContractBlockType=ContractGuaranteeBlock}
      mask init:
      | set_param(gcb, 'LinkStatus', 'none');
      mask DialogControl DescTextVar Prompt: Guarantee block
  EUL_006_3 : Subsystem  TreatAsAtomicUnit=on  mask(ContractGuaranteeBlock){ContractBlockType=ContractGuaranteeBlock}
      mask init:
      | set_param(gcb, 'LinkStatus', 'none');
      mask DialogControl DescTextVar Prompt: Guarantee block
  EUL_006_4 : Subsystem  TreatAsAtomicUnit=on  mask(ContractGuaranteeBlock){ContractBlockType=ContractGuaranteeBlock}
      mask init:
      | set_param(gcb, 'LinkStatus', 'none');
      mask DialogControl DescTextVar Prompt: Guarantee block
  EUL_007 : Subsystem  TreatAsAtomicUnit=on  mask(ContractGuaranteeBlock){ContractBlockType=ContractGuaranteeBlock}
      mask init:
      | set_param(gcb, 'LinkStatus', 'none');
      mask DialogControl DescTextVar Prompt: Guarantee block
  EUL_008 : Subsystem  TreatAsAtomicUnit=on  mask(ContractGuaranteeBlock){ContractBlockType=ContractGuaranteeBlock}
      mask init:
      | set_param(gcb, 'LinkStatus', 'none');
      mask DialogControl DescTextVar Prompt: Guarantee block
  Reshape : Reshape
  abs_call : Subsystem  TreatAsAtomicUnit=on
  c1xc1Transpose_operator : Sum  OutDataTypeStr=double
  c1xc2Transpose_operator : Sum  OutDataTypeStr=double
  c1xc3Transpose_operator : Sum  OutDataTypeStr=double
  c2xc2Transpose_operator : Sum  OutDataTypeStr=double
  c2xc3Transpose_operator : Sum  OutDataTypeStr=double
  c3xc3Transpose_operator : Sum  OutDataTypeStr=double
  det_3x3_call : Subsystem  TreatAsAtomicUnit=on
  r1xr1Transpose_operator : Sum  OutDataTypeStr=double
  r1xr2Transpose_operator : Sum  OutDataTypeStr=double
  r1xr3Transpose_operator : Sum  OutDataTypeStr=double
  r2xr1Transpose_operator : Sum  OutDataTypeStr=double
  r2xr2Transpose_operator : Sum  OutDataTypeStr=double
  r2xr3Transpose_operator : Sum  OutDataTypeStr=double
  r3xr1Transpose_operator : Sum  OutDataTypeStr=double
  r3xr2Transpose_operator : Sum  OutDataTypeStr=double
  r3xr3Transpose_operator : Sum  OutDataTypeStr=double
  spec113_operator : RelationalOperator  Operator===  OutDataTypeStr=boolean  RndMeth=Simplest
  spec123_operator : RelationalOperator  Operator===  OutDataTypeStr=boolean  RndMeth=Simplest
  spec145_operator : RelationalOperator  Operator===  OutDataTypeStr=boolean  RndMeth=Simplest
  spec169_operator : RelationalOperator  Operator===  OutDataTypeStr=boolean  RndMeth=Simplest
  spec177_operator : RelationalOperator  Operator===  OutDataTypeStr=boolean  RndMeth=Simplest
  spec187_operator : RelationalOperator  Operator===  OutDataTypeStr=boolean  RndMeth=Simplest
  spec197_operator : RelationalOperator  Operator===  OutDataTypeStr=boolean  RndMeth=Simplest
  spec217_operator : RelationalOperator  Operator===  OutDataTypeStr=boolean  RndMeth=Simplest
  spec237_operator : RelationalOperator  Operator===  OutDataTypeStr=boolean  RndMeth=Simplest
  spec257_operator : RelationalOperator  Operator===  OutDataTypeStr=boolean  RndMeth=Simplest
  spec292_operator : RelationalOperator  Operator===  OutDataTypeStr=boolean  RndMeth=Simplest
  spec319_operator : Subsystem  TreatAsAtomicUnit=on
  spec432_operator : Logic  AllPortsSameDT=off  OutDataTypeStr=boolean
  spec449_operator : Logic  AllPortsSameDT=off  OutDataTypeStr=boolean
  spec466_operator : Logic  AllPortsSameDT=off  OutDataTypeStr=boolean
  spec483_operator : Logic  AllPortsSameDT=off  OutDataTypeStr=boolean
  spec67_operator : RelationalOperator  Operator===  OutDataTypeStr=boolean  RndMeth=Simplest
  spec689_operator : Logic  AllPortsSameDT=off  OutDataTypeStr=boolean
  spec694_operator : RelationalOperator  Operator===  OutDataTypeStr=boolean  RndMeth=Simplest
  spec694_rhs_2 : Constant  Value=1.0  OutDataTypeStr=double
  spec91_operator : RelationalOperator  Operator===  OutDataTypeStr=boolean  RndMeth=Simplest
  validator : M-S-Function  LoadFcn=saveValidatorParameters(gcb);  InitFcn=contractBeforeSimulation();  StopFcn=contractAfterSimulation();  FunctionName=contract  mask(ContractValidatorBlock){assumePorts=0, guaranteePorts=20, modePorts=0, ContractBlockType=ContractValidatorBlock, createInportsCheckbox=off}
      mask prompts: assumePorts "Assume ports     :"; guaranteePorts "Guarantee ports :"; modePorts "Mode ports        :"; createInportsCheckbox "Create inports and connect them automatically"
      mask init:
      | set_param(gcb,'LinkStatus','none');
      | contract_callback('inputs_callback',gcb);
      mask DialogControl DescTextVar Prompt: The validator block implements the following logic: <br> <br> <b>Sofar</b>(assume<sub>1</sub> <b>&#8743;</b> assume<sub>2</sub> <b>&#8743;</b> ... assume<sub>k</sub>) <b>&rarr;</b> (guarantee<sub>1</sub> <b>&#8743;</b> guarantee<sub>2</sub> <b>&#8743;</b> ... guarantee<sub>m</sub> <b>&#8743;</b>  mode<sub>1</sub> <b>&#8743;</b> mode<sub>2</sub> <b>&#8743;</b> ... <b>&#8743;</b> mode<sub>n</sub> )<br> where mode<sub>i</sub> = require<sub>i</sub> <b>&rarr;</b> ensure<sub>i</sub>
      mask Display:
      | color('black');
      | port_label('input',1,'guarantee');
      | port_label('input',2,'guarantee');
      | port_label('input',3,'guarantee');
      | port_label('input',4,'guarantee');
      | port_label('input',5,'guarantee');
      | port_label('input',6,'guarantee');
      | port_label('input',7,'guarantee');
      | port_label('input',8,'guarantee');
      | port_label('input',9,'guarantee');
      | port_label('input',10,'guarantee');
      | port_label('input',11,'guarantee');
      | port_label('input',12,'guarantee');
      | port_label('input',13,'guarantee');
      | port_label('input',14,'guarantee');
      | port_label('input',15,'guarantee');
      | port_label('input',16,'guarantee');
      | port_label('input',17,'guarantee');
      | port_label('input',18,'guarantee');
      | port_label('input',19,'guarantee');
      | port_label('input',20,'guarantee');
      | port_label('output',1,'valid');
  xxeuler321_Spec_100_operator : Sum  OutDataTypeStr=double
  xxeuler321_Spec_101_cos_call : Trigonometry  Operator=cos
  xxeuler321_Spec_102_sin_call : Trigonometry
  xxeuler321_Spec_103_sin_call : Trigonometry
  xxeuler321_Spec_104_operator : Product  OutDataTypeStr=double
  xxeuler321_Spec_105_operator : Product  OutDataTypeStr=double
  xxeuler321_Spec_106_sin_call : Trigonometry
  xxeuler321_Spec_107_cos_call : Trigonometry  Operator=cos
  xxeuler321_Spec_108_operator : Gain  Gain=-1  OutDataTypeStr=double
  xxeuler321_Spec_109_operator : Product  OutDataTypeStr=double
  xxeuler321_Spec_10_operator : Logic  AllPortsSameDT=off  OutDataTypeStr=boolean
  xxeuler321_Spec_110_operator : Sum  OutDataTypeStr=double
  xxeuler321_Spec_111_cos_call : Trigonometry  Operator=cos
  xxeuler321_Spec_112_cos_call : Trigonometry  Operator=cos
  xxeuler321_Spec_113_operator : Product  OutDataTypeStr=double
  xxeuler321_Spec_114_rhs : Constant  Value=3.1415926536  OutDataTypeStr=double
  xxeuler321_Spec_115_operator : Product  OutDataTypeStr=double
  xxeuler321_Spec_116_operator : Product  OutDataTypeStr=double
  xxeuler321_Spec_117_operator : Product  OutDataTypeStr=double
  xxeuler321_Spec_118_operator : Sum  OutDataTypeStr=double
  xxeuler321_Spec_119_operator : Product  OutDataTypeStr=double
  xxeuler321_Spec_11_operator : Logic  AllPortsSameDT=off  OutDataTypeStr=boolean
  xxeuler321_Spec_120_operator : Product  OutDataTypeStr=double
  xxeuler321_Spec_121_operator : Product  OutDataTypeStr=double
  xxeuler321_Spec_122_operator : Sum  OutDataTypeStr=double
  xxeuler321_Spec_123_operator : Product  OutDataTypeStr=double
  xxeuler321_Spec_124_operator : Product  OutDataTypeStr=double
  xxeuler321_Spec_125_operator : Product  OutDataTypeStr=double
  xxeuler321_Spec_126_operator : Sum  OutDataTypeStr=double
  xxeuler321_Spec_127_operator : Product  OutDataTypeStr=double
  xxeuler321_Spec_128_operator : Product  OutDataTypeStr=double
  xxeuler321_Spec_129_operator : Product  OutDataTypeStr=double
  xxeuler321_Spec_12_operator : Logic  AllPortsSameDT=off  OutDataTypeStr=boolean
  xxeuler321_Spec_130_operator : Sum  OutDataTypeStr=double
  xxeuler321_Spec_131_operator : Product  OutDataTypeStr=double
  xxeuler321_Spec_132_operator : Product  OutDataTypeStr=double
  xxeuler321_Spec_133_operator : Product  OutDataTypeStr=double
  xxeuler321_Spec_134_operator : Sum  OutDataTypeStr=double
  xxeuler321_Spec_135_operator : Product  OutDataTypeStr=double
  xxeuler321_Spec_136_operator : Product  OutDataTypeStr=double
  xxeuler321_Spec_137_operator : Product  OutDataTypeStr=double
  xxeuler321_Spec_138_operator : Sum  OutDataTypeStr=double
  xxeuler321_Spec_139_operator : Sum  OutDataTypeStr=double
  xxeuler321_Spec_13_operator : Logic  AllPortsSameDT=off  OutDataTypeStr=boolean
  xxeuler321_Spec_140_operator : Product  OutDataTypeStr=double
  xxeuler321_Spec_141_operator : Product  OutDataTypeStr=double
  xxeuler321_Spec_142_operator : Product  OutDataTypeStr=double
  xxeuler321_Spec_143_operator : Sum  OutDataTypeStr=double
  xxeuler321_Spec_144_operator : Product  OutDataTypeStr=double
  xxeuler321_Spec_145_operator : Product  OutDataTypeStr=double
  xxeuler321_Spec_146_operator : Product  OutDataTypeStr=double
  xxeuler321_Spec_147_operator : Sum  OutDataTypeStr=double
  xxeuler321_Spec_148_operator : Product  OutDataTypeStr=double
  xxeuler321_Spec_149_operator : Product  OutDataTypeStr=double
  xxeuler321_Spec_14_operator : Logic  AllPortsSameDT=off  OutDataTypeStr=boolean
  xxeuler321_Spec_150_operator : Product  OutDataTypeStr=double
  xxeuler321_Spec_151_operator : Sum  OutDataTypeStr=double
  xxeuler321_Spec_152_operator : Sum  OutDataTypeStr=double
  xxeuler321_Spec_153_operator : Product  OutDataTypeStr=double
  xxeuler321_Spec_154_operator : Product  OutDataTypeStr=double
  xxeuler321_Spec_155_operator : Product  OutDataTypeStr=double
  xxeuler321_Spec_156_operator : Sum  OutDataTypeStr=double
  xxeuler321_Spec_157_operator : Product  OutDataTypeStr=double
  xxeuler321_Spec_158_operator : Product  OutDataTypeStr=double
  xxeuler321_Spec_159_operator : Product  OutDataTypeStr=double
  xxeuler321_Spec_15_operator : Logic  AllPortsSameDT=off  OutDataTypeStr=boolean
  xxeuler321_Spec_160_operator : Sum  OutDataTypeStr=double
  xxeuler321_Spec_161_operator : Product  OutDataTypeStr=double
  xxeuler321_Spec_162_operator : Product  OutDataTypeStr=double
  xxeuler321_Spec_163_operator : Product  OutDataTypeStr=double
  xxeuler321_Spec_164_operator : Sum  OutDataTypeStr=double
  xxeuler321_Spec_165_operator : Sum  OutDataTypeStr=double
  xxeuler321_Spec_16_operator : Logic  AllPortsSameDT=off  OutDataTypeStr=boolean
  xxeuler321_Spec_17_operator : RelationalOperator  Operator===  OutDataTypeStr=boolean  RndMeth=Simplest
  xxeuler321_Spec_17_rhs_2 : Constant  Value=0.0  OutDataTypeStr=double
  xxeuler321_Spec_18_operator : RelationalOperator  Operator===  OutDataTypeStr=boolean  RndMeth=Simplest
  xxeuler321_Spec_18_rhs_2 : Constant  Value=0.0  OutDataTypeStr=double
  xxeuler321_Spec_19_operator : RelationalOperator  Operator===  OutDataTypeStr=boolean  RndMeth=Simplest
  xxeuler321_Spec_19_rhs_2 : Constant  Value=0.0  OutDataTypeStr=double
  xxeuler321_Spec_1_operator : RelationalOperator  Operator===  OutDataTypeStr=boolean  RndMeth=Simplest
  xxeuler321_Spec_1_rhs_2 : Constant  Value=1.0  OutDataTypeStr=double
  xxeuler321_Spec_20_operator : Logic  AllPortsSameDT=off  OutDataTypeStr=boolean
  xxeuler321_Spec_21_operator : RelationalOperator  Operator===  OutDataTypeStr=boolean  RndMeth=Simplest
  xxeuler321_Spec_21_rhs_2 : Constant  Value=1.0  OutDataTypeStr=double
  xxeuler321_Spec_22_operator : RelationalOperator  Operator===  OutDataTypeStr=boolean  RndMeth=Simplest
  xxeuler321_Spec_22_rhs_2 : Constant  Value=1.0  OutDataTypeStr=double
  xxeuler321_Spec_23_operator : RelationalOperator  Operator===  OutDataTypeStr=boolean  RndMeth=Simplest
  xxeuler321_Spec_23_rhs_2 : Constant  Value=1.0  OutDataTypeStr=double
  xxeuler321_Spec_24_operator : Logic  AllPortsSameDT=off  OutDataTypeStr=boolean
  xxeuler321_Spec_25_operator : RelationalOperator  Operator===  OutDataTypeStr=boolean  RndMeth=Simplest
  xxeuler321_Spec_25_rhs_2 : Constant  Value=0.0  OutDataTypeStr=double
  xxeuler321_Spec_26_operator : RelationalOperator  Operator===  OutDataTypeStr=boolean  RndMeth=Simplest
  xxeuler321_Spec_26_rhs_2 : Constant  Value=0.0  OutDataTypeStr=double
  xxeuler321_Spec_27_operator : RelationalOperator  Operator===  OutDataTypeStr=boolean  RndMeth=Simplest
  xxeuler321_Spec_27_rhs_2 : Constant  Value=0.0  OutDataTypeStr=double
  xxeuler321_Spec_28_operator : Logic  AllPortsSameDT=off  OutDataTypeStr=boolean
  xxeuler321_Spec_29_operator : RelationalOperator  Operator===  OutDataTypeStr=boolean  RndMeth=Simplest
  xxeuler321_Spec_29_rhs_2 : Constant  Value=1.0  OutDataTypeStr=double
  xxeuler321_Spec_2_operator : RelationalOperator  Operator===  OutDataTypeStr=boolean  RndMeth=Simplest
  xxeuler321_Spec_2_rhs_2 : Constant  Value=0.0  OutDataTypeStr=double
  xxeuler321_Spec_30_operator : RelationalOperator  Operator===  OutDataTypeStr=boolean  RndMeth=Simplest
  xxeuler321_Spec_30_rhs_2 : Constant  Value=1.0  OutDataTypeStr=double
  xxeuler321_Spec_31_operator : RelationalOperator  Operator===  OutDataTypeStr=boolean  RndMeth=Simplest
  xxeuler321_Spec_31_rhs_2 : Constant  Value=1.0  OutDataTypeStr=double
  xxeuler321_Spec_32_operator : Logic  AllPortsSameDT=off  OutDataTypeStr=boolean
  xxeuler321_Spec_33_operator : RelationalOperator  Operator=~=  OutDataTypeStr=boolean  RndMeth=Simplest
  xxeuler321_Spec_33_rhs_2 : Constant  Value=0.0  OutDataTypeStr=double
  xxeuler321_Spec_34_operator : Product  Inputs=*/  OutDataTypeStr=double
  xxeuler321_Spec_34_rhs_2 : Constant  Value=2.0  OutDataTypeStr=double
  xxeuler321_Spec_36_operator : RelationalOperator  Operator=~=  OutDataTypeStr=boolean  RndMeth=Simplest
  xxeuler321_Spec_37_operator : Product  OutDataTypeStr=double
  xxeuler321_Spec_38_operator : Product  OutDataTypeStr=double
  xxeuler321_Spec_39_operator : Product  OutDataTypeStr=double
  xxeuler321_Spec_3_operator : RelationalOperator  Operator===  OutDataTypeStr=boolean  RndMeth=Simplest
  xxeuler321_Spec_3_rhs_2 : Constant  Value=0.0  OutDataTypeStr=double
  xxeuler321_Spec_40_operator : Sum  OutDataTypeStr=double
  xxeuler321_Spec_41_operator : Sum  OutDataTypeStr=double
  xxeuler321_Spec_42_operator : Product  OutDataTypeStr=double
  xxeuler321_Spec_43_operator : Product  OutDataTypeStr=double
  xxeuler321_Spec_44_operator : Product  OutDataTypeStr=double
  xxeuler321_Spec_45_operator : Sum  OutDataTypeStr=double
  xxeuler321_Spec_46_operator : Sum  OutDataTypeStr=double
  xxeuler321_Spec_47_operator : Product  OutDataTypeStr=double
  xxeuler321_Spec_48_operator : Product  OutDataTypeStr=double
  xxeuler321_Spec_49_operator : Product  OutDataTypeStr=double
  xxeuler321_Spec_4_operator : RelationalOperator  Operator===  OutDataTypeStr=boolean  RndMeth=Simplest
  xxeuler321_Spec_4_rhs_2 : Constant  Value=0.0  OutDataTypeStr=double
  xxeuler321_Spec_50_operator : Sum  OutDataTypeStr=double
  xxeuler321_Spec_51_operator : Sum  OutDataTypeStr=double
  xxeuler321_Spec_52_operator : Product  OutDataTypeStr=double
  xxeuler321_Spec_53_operator : Product  OutDataTypeStr=double
  xxeuler321_Spec_54_operator : Product  OutDataTypeStr=double
  xxeuler321_Spec_55_operator : Sum  OutDataTypeStr=double
  xxeuler321_Spec_56_operator : Sum  OutDataTypeStr=double
  xxeuler321_Spec_57_operator : Product  OutDataTypeStr=double
  xxeuler321_Spec_58_operator : Product  OutDataTypeStr=double
  xxeuler321_Spec_59_operator : Product  OutDataTypeStr=double
  xxeuler321_Spec_5_operator : RelationalOperator  Operator===  OutDataTypeStr=boolean  RndMeth=Simplest
  xxeuler321_Spec_5_rhs_2 : Constant  Value=1.0  OutDataTypeStr=double
  xxeuler321_Spec_60_operator : Sum  OutDataTypeStr=double
  xxeuler321_Spec_61_operator : Sum  OutDataTypeStr=double
  xxeuler321_Spec_62_cos_call : Trigonometry  Operator=cos
  xxeuler321_Spec_63_cos_call : Trigonometry  Operator=cos
  xxeuler321_Spec_64_operator : Product  OutDataTypeStr=double
  xxeuler321_Spec_65_cos_call : Trigonometry  Operator=cos
  xxeuler321_Spec_66_sin_call : Trigonometry
  xxeuler321_Spec_67_operator : Product  OutDataTypeStr=double
  xxeuler321_Spec_68_sin_call : Trigonometry
  xxeuler321_Spec_69_operator : Gain  Gain=-1  OutDataTypeStr=double
  xxeuler321_Spec_6_operator : RelationalOperator  Operator===  OutDataTypeStr=boolean  RndMeth=Simplest
  xxeuler321_Spec_6_rhs_2 : Constant  Value=0.0  OutDataTypeStr=double
  xxeuler321_Spec_70_sin_call : Trigonometry
  xxeuler321_Spec_71_sin_call : Trigonometry
  xxeuler321_Spec_72_cos_call : Trigonometry  Operator=cos
  xxeuler321_Spec_73_operator : Product  OutDataTypeStr=double
  xxeuler321_Spec_74_operator : Product  OutDataTypeStr=double
  xxeuler321_Spec_75_cos_call : Trigonometry  Operator=cos
  xxeuler321_Spec_76_sin_call : Trigonometry
  xxeuler321_Spec_77_operator : Gain  Gain=-1  OutDataTypeStr=double
  xxeuler321_Spec_78_operator : Product  OutDataTypeStr=double
  xxeuler321_Spec_79_operator : Sum  OutDataTypeStr=double
  xxeuler321_Spec_7_operator : RelationalOperator  Operator===  OutDataTypeStr=boolean  RndMeth=Simplest
  xxeuler321_Spec_7_rhs_2 : Constant  Value=0.0  OutDataTypeStr=double
  xxeuler321_Spec_80_sin_call : Trigonometry
  xxeuler321_Spec_81_sin_call : Trigonometry
  xxeuler321_Spec_82_sin_call : Trigonometry
  xxeuler321_Spec_83_operator : Product  OutDataTypeStr=double
  xxeuler321_Spec_84_operator : Product  OutDataTypeStr=double
  xxeuler321_Spec_85_cos_call : Trigonometry  Operator=cos
  xxeuler321_Spec_86_cos_call : Trigonometry  Operator=cos
  xxeuler321_Spec_87_operator : Product  OutDataTypeStr=double
  xxeuler321_Spec_88_operator : Sum  OutDataTypeStr=double
  xxeuler321_Spec_89_sin_call : Trigonometry
  xxeuler321_Spec_8_operator : RelationalOperator  Operator===  OutDataTypeStr=boolean  RndMeth=Simplest
  xxeuler321_Spec_8_rhs_2 : Constant  Value=0.0  OutDataTypeStr=double
  xxeuler321_Spec_90_cos_call : Trigonometry  Operator=cos
  xxeuler321_Spec_91_operator : Product  OutDataTypeStr=double
  xxeuler321_Spec_92_cos_call : Trigonometry  Operator=cos
  xxeuler321_Spec_93_sin_call : Trigonometry
  xxeuler321_Spec_94_cos_call : Trigonometry  Operator=cos
  xxeuler321_Spec_95_operator : Product  OutDataTypeStr=double
  xxeuler321_Spec_96_operator : Product  OutDataTypeStr=double
  xxeuler321_Spec_97_sin_call : Trigonometry
  xxeuler321_Spec_98_sin_call : Trigonometry
  xxeuler321_Spec_99_operator : Product  OutDataTypeStr=double
  xxeuler321_Spec_9_operator : RelationalOperator  Operator===  OutDataTypeStr=boolean  RndMeth=Simplest
  xxeuler321_Spec_9_rhs_2 : Constant  Value=1.0  OutDataTypeStr=double
  valid : Outport
  wires:
  Demux1/1 -> xxeuler321_Spec_44_operator/1, xxeuler321_Spec_44_operator/2, spec217_operator/1
  Demux1/2 -> xxeuler321_Spec_43_operator/1, xxeuler321_Spec_43_operator/2, spec237_operator/1
  Demux1/3 -> spec257_operator/1, xxeuler321_Spec_42_operator/2, xxeuler321_Spec_42_operator/1
  Demux/3 -> xxeuler321_Spec_52_operator/2, xxeuler321_Spec_57_operator/2, xxeuler321_Spec_47_operator/2, xxeuler321_Spec_37_operator/2, xxeuler321_Spec_37_operator/1
  Demux/2 -> xxeuler321_Spec_53_operator/2, xxeuler321_Spec_58_operator/2, xxeuler321_Spec_48_operator/2, xxeuler321_Spec_38_operator/2, xxeuler321_Spec_38_operator/1
  Demux/1 -> xxeuler321_Spec_54_operator/2, xxeuler321_Spec_59_operator/2, xxeuler321_Spec_49_operator/2, xxeuler321_Spec_39_operator/2, xxeuler321_Spec_39_operator/1
  euler321_Spec_theta/1 -> abs_call/1(abs_x), xxeuler321_Spec_112_cos_call/1, xxeuler321_Spec_90_cos_call/1, xxeuler321_Spec_93_sin_call/1, xxeuler321_Spec_81_sin_call/1, xxeuler321_Spec_71_sin_call/1, xxeuler321_Spec_68_sin_call/1, xxeuler321_Spec_65_cos_call/1, xxeuler321_Spec_62_cos_call/1, xxeuler321_Spec_102_sin_call/1
  xxeuler321_Spec_115_operator/1 -> c1xc1Transpose_operator/2, xxeuler321_Spec_165_operator/1
  xxeuler321_Spec_116_operator/1 -> xxeuler321_Spec_118_operator/2, xxeuler321_Spec_152_operator/1
  xxeuler321_Spec_117_operator/1 -> xxeuler321_Spec_118_operator/1, xxeuler321_Spec_139_operator/1
  xxeuler321_Spec_119_operator/1 -> c2xc2Transpose_operator/2, xxeuler321_Spec_165_operator/2
  xxeuler321_Spec_120_operator/1 -> xxeuler321_Spec_122_operator/2, xxeuler321_Spec_152_operator/2
  xxeuler321_Spec_121_operator/1 -> xxeuler321_Spec_122_operator/1, xxeuler321_Spec_139_operator/2
  xxeuler321_Spec_123_operator/1 -> c3xc3Transpose_operator/2, r3xr3Transpose_operator/2
  r3xr3Transpose_operator/1 -> xxeuler321_Spec_1_operator/1, xxeuler321_Spec_29_operator/1
  r2xr3Transpose_operator/1 -> xxeuler321_Spec_25_operator/1, xxeuler321_Spec_4_operator/1
  r2xr2Transpose_operator/1 -> xxeuler321_Spec_30_operator/1, xxeuler321_Spec_5_operator/1
  r1xr3Transpose_operator/1 -> xxeuler321_Spec_26_operator/1, xxeuler321_Spec_7_operator/1
  r1xr2Transpose_operator/1 -> xxeuler321_Spec_27_operator/1, xxeuler321_Spec_8_operator/1
  r1xr1Transpose_operator/1 -> xxeuler321_Spec_31_operator/1, xxeuler321_Spec_9_operator/1
  xxeuler321_Spec_125_operator/1 -> r1xr1Transpose_operator/2, xxeuler321_Spec_126_operator/1
  xxeuler321_Spec_124_operator/1 -> r2xr2Transpose_operator/2, xxeuler321_Spec_126_operator/2
  det_3x3_call/1(det_3x3_det) -> spec694_operator/1, xxeuler321_Spec_33_operator/1
  Demux3/9 -> xxeuler321_Spec_144_operator/2, xxeuler321_Spec_153_operator/2, xxeuler321_Spec_157_operator/1, xxeuler321_Spec_161_operator/1, xxeuler321_Spec_123_operator/2, xxeuler321_Spec_123_operator/1, xxeuler321_Spec_131_operator/2, xxeuler321_Spec_135_operator/2, spec197_operator/1, xxeuler321_Spec_47_operator/1, det_3x3_call/9(det_3x3_a33)
  Demux3/8 -> xxeuler321_Spec_140_operator/2, xxeuler321_Spec_148_operator/1, xxeuler321_Spec_124_operator/2, xxeuler321_Spec_124_operator/1, xxeuler321_Spec_153_operator/1, xxeuler321_Spec_161_operator/2, xxeuler321_Spec_132_operator/2, xxeuler321_Spec_136_operator/2, spec187_operator/1, xxeuler321_Spec_52_operator/1, det_3x3_call/8(det_3x3_a23)
  Demux3/7 -> xxeuler321_Spec_125_operator/1, xxeuler321_Spec_125_operator/2, xxeuler321_Spec_140_operator/1, xxeuler321_Spec_144_operator/1, xxeuler321_Spec_148_operator/2, xxeuler321_Spec_157_operator/2, xxeuler321_Spec_133_operator/2, xxeuler321_Spec_137_operator/2, spec177_operator/1, xxeuler321_Spec_57_operator/1, det_3x3_call/7(det_3x3_a13)
  Demux3/6 -> xxeuler321_Spec_145_operator/2, xxeuler321_Spec_154_operator/2, xxeuler321_Spec_158_operator/1, xxeuler321_Spec_162_operator/1, xxeuler321_Spec_119_operator/2, xxeuler321_Spec_119_operator/1, xxeuler321_Spec_127_operator/2, xxeuler321_Spec_135_operator/1, spec169_operator/1, xxeuler321_Spec_48_operator/1, det_3x3_call/6(det_3x3_a32)
  Demux3/5 -> xxeuler321_Spec_141_operator/2, xxeuler321_Spec_149_operator/1, xxeuler321_Spec_120_operator/2, xxeuler321_Spec_120_operator/1, xxeuler321_Spec_154_operator/1, xxeuler321_Spec_162_operator/2, xxeuler321_Spec_128_operator/2, xxeuler321_Spec_136_operator/1, spec145_operator/1, xxeuler321_Spec_53_operator/1, det_3x3_call/5(det_3x3_a22)
  Demux3/4 -> xxeuler321_Spec_121_operator/1, xxeuler321_Spec_121_operator/2, xxeuler321_Spec_141_operator/1, xxeuler321_Spec_145_operator/1, xxeuler321_Spec_149_operator/2, xxeuler321_Spec_158_operator/2, xxeuler321_Spec_129_operator/2, xxeuler321_Spec_137_operator/1, spec123_operator/1, xxeuler321_Spec_58_operator/1, det_3x3_call/4(det_3x3_a12)
  Demux3/3 -> xxeuler321_Spec_146_operator/2, xxeuler321_Spec_155_operator/2, xxeuler321_Spec_159_operator/1, xxeuler321_Spec_163_operator/1, xxeuler321_Spec_115_operator/2, xxeuler321_Spec_115_operator/1, xxeuler321_Spec_127_operator/1, xxeuler321_Spec_131_operator/1, spec113_operator/1, xxeuler321_Spec_49_operator/1, det_3x3_call/3(det_3x3_a31)
  Demux3/2 -> xxeuler321_Spec_142_operator/2, xxeuler321_Spec_150_operator/1, xxeuler321_Spec_116_operator/2, xxeuler321_Spec_116_operator/1, xxeuler321_Spec_155_operator/1, xxeuler321_Spec_163_operator/2, spec91_operator/1, xxeuler321_Spec_128_operator/1, xxeuler321_Spec_132_operator/1, xxeuler321_Spec_54_operator/1, det_3x3_call/2(det_3x3_a21)
  Demux3/1 -> xxeuler321_Spec_117_operator/1, xxeuler321_Spec_117_operator/2, xxeuler321_Spec_142_operator/1, xxeuler321_Spec_146_operator/1, xxeuler321_Spec_150_operator/2, xxeuler321_Spec_159_operator/2, xxeuler321_Spec_129_operator/1, xxeuler321_Spec_133_operator/1, spec67_operator/1, xxeuler321_Spec_59_operator/1, det_3x3_call/1(det_3x3_a11)
  euler321_Spec_psi/1 -> xxeuler321_Spec_101_cos_call/1, xxeuler321_Spec_106_sin_call/1, xxeuler321_Spec_92_cos_call/1, xxeuler321_Spec_97_sin_call/1, xxeuler321_Spec_89_sin_call/1, xxeuler321_Spec_80_sin_call/1, xxeuler321_Spec_85_cos_call/1, xxeuler321_Spec_70_sin_call/1, xxeuler321_Spec_75_cos_call/1, xxeuler321_Spec_111_cos_call/1
  euler321_Spec_phi/1 -> xxeuler321_Spec_103_sin_call/1, xxeuler321_Spec_107_cos_call/1, xxeuler321_Spec_94_cos_call/1, xxeuler321_Spec_98_sin_call/1, xxeuler321_Spec_82_sin_call/1, xxeuler321_Spec_86_cos_call/1, xxeuler321_Spec_72_cos_call/1, xxeuler321_Spec_76_sin_call/1, xxeuler321_Spec_66_sin_call/1, xxeuler321_Spec_63_cos_call/1
  Vi/1 -> Demux/1
  Vb/1 -> Demux1/1
  Reshape/1 -> Demux3/1
  DCM321/1 -> Reshape/1
  xxeuler321_Spec_118_operator/1 -> c1xc1Transpose_operator/1
  xxeuler321_Spec_130_operator/1 -> c1xc2Transpose_operator/1
  xxeuler321_Spec_127_operator/1 -> c1xc2Transpose_operator/2
  xxeuler321_Spec_134_operator/1 -> c1xc3Transpose_operator/1
  xxeuler321_Spec_131_operator/1 -> c1xc3Transpose_operator/2
  xxeuler321_Spec_122_operator/1 -> c2xc2Transpose_operator/1
  xxeuler321_Spec_138_operator/1 -> c2xc3Transpose_operator/1
  xxeuler321_Spec_135_operator/1 -> c2xc3Transpose_operator/2
  xxeuler321_Spec_126_operator/1 -> c3xc3Transpose_operator/1
  spec67_operator/1 -> EUL_001_1/1(In1)
  spec91_operator/1 -> EUL_001_2/1(In1)
  spec113_operator/1 -> EUL_001_3/1(In1)
  spec123_operator/1 -> EUL_001_4/1(In1)
  spec145_operator/1 -> EUL_001_5/1(In1)
  spec169_operator/1 -> EUL_001_6/1(In1)
  spec177_operator/1 -> EUL_001_7/1(In1)
  spec187_operator/1 -> EUL_001_8/1(In1)
  spec197_operator/1 -> EUL_001_9/1(In1)
  spec217_operator/1 -> EUL_002_1/1(In1)
  spec237_operator/1 -> EUL_002_2/1(In1)
  spec257_operator/1 -> EUL_002_3/1(In1)
  spec292_operator/1 -> EUL_003/1(In1)
  spec319_operator/1(A_equal__equal__gt_B) -> EUL_004/1(In1)
  spec432_operator/1 -> EUL_006_1/1(In1)
  spec449_operator/1 -> EUL_006_2/1(In1)
  spec466_operator/1 -> EUL_006_3/1(In1)
  spec483_operator/1 -> EUL_006_4/1(In1)
  spec689_operator/1 -> EUL_007/1(In1)
  spec694_operator/1 -> EUL_008/1(In1)
  xxeuler321_Spec_139_operator/1 -> r1xr1Transpose_operator/1
  xxeuler321_Spec_143_operator/1 -> r1xr2Transpose_operator/1
  xxeuler321_Spec_140_operator/1 -> r1xr2Transpose_operator/2
  xxeuler321_Spec_147_operator/1 -> r1xr3Transpose_operator/1
  xxeuler321_Spec_144_operator/1 -> r1xr3Transpose_operator/2
  xxeuler321_Spec_151_operator/1 -> r2xr1Transpose_operator/1
  xxeuler321_Spec_148_operator/1 -> r2xr1Transpose_operator/2
  xxeuler321_Spec_152_operator/1 -> r2xr2Transpose_operator/1
  xxeuler321_Spec_156_operator/1 -> r2xr3Transpose_operator/1
  xxeuler321_Spec_153_operator/1 -> r2xr3Transpose_operator/2
  xxeuler321_Spec_160_operator/1 -> r3xr1Transpose_operator/1
  xxeuler321_Spec_157_operator/1 -> r3xr1Transpose_operator/2
  xxeuler321_Spec_164_operator/1 -> r3xr2Transpose_operator/1
  xxeuler321_Spec_161_operator/1 -> r3xr2Transpose_operator/2
  xxeuler321_Spec_165_operator/1 -> r3xr3Transpose_operator/1
  xxeuler321_Spec_100_operator/1 -> spec113_operator/2
  xxeuler321_Spec_91_operator/1 -> spec123_operator/2
  xxeuler321_Spec_88_operator/1 -> spec145_operator/2
  xxeuler321_Spec_79_operator/1 -> spec169_operator/2
  xxeuler321_Spec_69_operator/1 -> spec177_operator/2
  xxeuler321_Spec_67_operator/1 -> spec187_operator/2
  xxeuler321_Spec_64_operator/1 -> spec197_operator/2
  xxeuler321_Spec_61_operator/1 -> spec217_operator/2
  xxeuler321_Spec_56_operator/1 -> spec237_operator/2
  xxeuler321_Spec_51_operator/1 -> spec257_operator/2
  xxeuler321_Spec_46_operator/1 -> spec292_operator/1
  xxeuler321_Spec_41_operator/1 -> spec292_operator/2
  xxeuler321_Spec_36_operator/1 -> spec319_operator/1(A)
  xxeuler321_Spec_33_operator/1 -> spec319_operator/2(B)
  xxeuler321_Spec_32_operator/1 -> spec432_operator/1
  xxeuler321_Spec_29_operator/1 -> spec432_operator/2
  xxeuler321_Spec_28_operator/1 -> spec449_operator/1
  xxeuler321_Spec_25_operator/1 -> spec449_operator/2
  xxeuler321_Spec_24_operator/1 -> spec466_operator/1
  xxeuler321_Spec_21_operator/1 -> spec466_operator/2
  xxeuler321_Spec_20_operator/1 -> spec483_operator/1
  xxeuler321_Spec_17_operator/1 -> spec483_operator/2
  xxeuler321_Spec_113_operator/1 -> spec67_operator/2
  xxeuler321_Spec_16_operator/1 -> spec689_operator/1
  xxeuler321_Spec_1_operator/1 -> spec689_operator/2
  spec694_rhs_2/1 -> spec694_operator/2
  xxeuler321_Spec_110_operator/1 -> spec91_operator/2
  EUL_001_1/1(guarantee) -> validator/1
  EUL_001_2/1(guarantee) -> validator/2
  EUL_001_3/1(guarantee) -> validator/3
  EUL_001_4/1(guarantee) -> validator/4
  EUL_001_5/1(guarantee) -> validator/5
  EUL_001_6/1(guarantee) -> validator/6
  EUL_001_7/1(guarantee) -> validator/7
  EUL_001_8/1(guarantee) -> validator/8
  EUL_001_9/1(guarantee) -> validator/9
  EUL_002_1/1(guarantee) -> validator/10
  EUL_002_2/1(guarantee) -> validator/11
  EUL_002_3/1(guarantee) -> validator/12
  EUL_003/1(guarantee) -> validator/13
  EUL_004/1(guarantee) -> validator/14
  EUL_006_1/1(guarantee) -> validator/15
  EUL_006_2/1(guarantee) -> validator/16
  EUL_006_3/1(guarantee) -> validator/17
  EUL_006_4/1(guarantee) -> validator/18
  EUL_007/1(guarantee) -> validator/19
  EUL_008/1(guarantee) -> validator/20
  xxeuler321_Spec_99_operator/1 -> xxeuler321_Spec_100_operator/1
  xxeuler321_Spec_96_operator/1 -> xxeuler321_Spec_100_operator/2
  xxeuler321_Spec_103_sin_call/1 -> xxeuler321_Spec_104_operator/1
  xxeuler321_Spec_102_sin_call/1 -> xxeuler321_Spec_104_operator/2
  xxeuler321_Spec_104_operator/1 -> xxeuler321_Spec_105_operator/1
  xxeuler321_Spec_101_cos_call/1 -> xxeuler321_Spec_105_operator/2
  xxeuler321_Spec_107_cos_call/1 -> xxeuler321_Spec_108_operator/1
  xxeuler321_Spec_108_operator/1 -> xxeuler321_Spec_109_operator/1
  xxeuler321_Spec_106_sin_call/1 -> xxeuler321_Spec_109_operator/2
  xxeuler321_Spec_9_operator/1 -> xxeuler321_Spec_10_operator/1
  xxeuler321_Spec_8_operator/1 -> xxeuler321_Spec_10_operator/2
  xxeuler321_Spec_109_operator/1 -> xxeuler321_Spec_110_operator/1
  xxeuler321_Spec_105_operator/1 -> xxeuler321_Spec_110_operator/2
  xxeuler321_Spec_112_cos_call/1 -> xxeuler321_Spec_113_operator/1
  xxeuler321_Spec_111_cos_call/1 -> xxeuler321_Spec_113_operator/2
  xxeuler321_Spec_10_operator/1 -> xxeuler321_Spec_11_operator/1
  xxeuler321_Spec_7_operator/1 -> xxeuler321_Spec_11_operator/2
  xxeuler321_Spec_11_operator/1 -> xxeuler321_Spec_12_operator/1
  xxeuler321_Spec_6_operator/1 -> xxeuler321_Spec_12_operator/2
  xxeuler321_Spec_129_operator/1 -> xxeuler321_Spec_130_operator/1
  xxeuler321_Spec_128_operator/1 -> xxeuler321_Spec_130_operator/2
  xxeuler321_Spec_133_operator/1 -> xxeuler321_Spec_134_operator/1
  xxeuler321_Spec_132_operator/1 -> xxeuler321_Spec_134_operator/2
  xxeuler321_Spec_137_operator/1 -> xxeuler321_Spec_138_operator/1
  xxeuler321_Spec_136_operator/1 -> xxeuler321_Spec_138_operator/2
  xxeuler321_Spec_12_operator/1 -> xxeuler321_Spec_13_operator/1
  xxeuler321_Spec_5_operator/1 -> xxeuler321_Spec_13_operator/2
  xxeuler321_Spec_142_operator/1 -> xxeuler321_Spec_143_operator/1
  xxeuler321_Spec_141_operator/1 -> xxeuler321_Spec_143_operator/2
  xxeuler321_Spec_146_operator/1 -> xxeuler321_Spec_147_operator/1
  xxeuler321_Spec_145_operator/1 -> xxeuler321_Spec_147_operator/2
  xxeuler321_Spec_13_operator/1 -> xxeuler321_Spec_14_operator/1
  xxeuler321_Spec_4_operator/1 -> xxeuler321_Spec_14_operator/2
  xxeuler321_Spec_150_operator/1 -> xxeuler321_Spec_151_operator/1
  xxeuler321_Spec_149_operator/1 -> xxeuler321_Spec_151_operator/2
  xxeuler321_Spec_155_operator/1 -> xxeuler321_Spec_156_operator/1
  xxeuler321_Spec_154_operator/1 -> xxeuler321_Spec_156_operator/2
  xxeuler321_Spec_14_operator/1 -> xxeuler321_Spec_15_operator/1
  xxeuler321_Spec_3_operator/1 -> xxeuler321_Spec_15_operator/2
  xxeuler321_Spec_159_operator/1 -> xxeuler321_Spec_160_operator/1
  xxeuler321_Spec_158_operator/1 -> xxeuler321_Spec_160_operator/2
  xxeuler321_Spec_163_operator/1 -> xxeuler321_Spec_164_operator/1
  xxeuler321_Spec_162_operator/1 -> xxeuler321_Spec_164_operator/2
  xxeuler321_Spec_15_operator/1 -> xxeuler321_Spec_16_operator/1
  xxeuler321_Spec_2_operator/1 -> xxeuler321_Spec_16_operator/2
  c2xc3Transpose_operator/1 -> xxeuler321_Spec_17_operator/1
  xxeuler321_Spec_17_rhs_2/1 -> xxeuler321_Spec_17_operator/2
  c1xc3Transpose_operator/1 -> xxeuler321_Spec_18_operator/1
  xxeuler321_Spec_18_rhs_2/1 -> xxeuler321_Spec_18_operator/2
  c1xc2Transpose_operator/1 -> xxeuler321_Spec_19_operator/1
  xxeuler321_Spec_19_rhs_2/1 -> xxeuler321_Spec_19_operator/2
  xxeuler321_Spec_1_rhs_2/1 -> xxeuler321_Spec_1_operator/2
  xxeuler321_Spec_19_operator/1 -> xxeuler321_Spec_20_operator/1
  xxeuler321_Spec_18_operator/1 -> xxeuler321_Spec_20_operator/2
  c3xc3Transpose_operator/1 -> xxeuler321_Spec_21_operator/1
  xxeuler321_Spec_21_rhs_2/1 -> xxeuler321_Spec_21_operator/2
  c2xc2Transpose_operator/1 -> xxeuler321_Spec_22_operator/1
  xxeuler321_Spec_22_rhs_2/1 -> xxeuler321_Spec_22_operator/2
  c1xc1Transpose_operator/1 -> xxeuler321_Spec_23_operator/1
  xxeuler321_Spec_23_rhs_2/1 -> xxeuler321_Spec_23_operator/2
  xxeuler321_Spec_23_operator/1 -> xxeuler321_Spec_24_operator/1
  xxeuler321_Spec_22_operator/1 -> xxeuler321_Spec_24_operator/2
  xxeuler321_Spec_25_rhs_2/1 -> xxeuler321_Spec_25_operator/2
  xxeuler321_Spec_26_rhs_2/1 -> xxeuler321_Spec_26_operator/2
  xxeuler321_Spec_27_rhs_2/1 -> xxeuler321_Spec_27_operator/2
  xxeuler321_Spec_27_operator/1 -> xxeuler321_Spec_28_operator/1
  xxeuler321_Spec_26_operator/1 -> xxeuler321_Spec_28_operator/2
  xxeuler321_Spec_29_rhs_2/1 -> xxeuler321_Spec_29_operator/2
  r3xr2Transpose_operator/1 -> xxeuler321_Spec_2_operator/1
  xxeuler321_Spec_2_rhs_2/1 -> xxeuler321_Spec_2_operator/2
  xxeuler321_Spec_30_rhs_2/1 -> xxeuler321_Spec_30_operator/2
  xxeuler321_Spec_31_rhs_2/1 -> xxeuler321_Spec_31_operator/2
  xxeuler321_Spec_31_operator/1 -> xxeuler321_Spec_32_operator/1
  xxeuler321_Spec_30_operator/1 -> xxeuler321_Spec_32_operator/2
  xxeuler321_Spec_33_rhs_2/1 -> xxeuler321_Spec_33_operator/2
  xxeuler321_Spec_114_rhs/1 -> xxeuler321_Spec_34_operator/1
  xxeuler321_Spec_34_rhs_2/1 -> xxeuler321_Spec_34_operator/2
  abs_call/1(abs_y) -> xxeuler321_Spec_36_operator/1
  xxeuler321_Spec_34_operator/1 -> xxeuler321_Spec_36_operator/2
  r3xr1Transpose_operator/1 -> xxeuler321_Spec_3_operator/1
  xxeuler321_Spec_3_rhs_2/1 -> xxeuler321_Spec_3_operator/2
  xxeuler321_Spec_39_operator/1 -> xxeuler321_Spec_40_operator/1
  xxeuler321_Spec_38_operator/1 -> xxeuler321_Spec_40_operator/2
  xxeuler321_Spec_40_operator/1 -> xxeuler321_Spec_41_operator/1
  xxeuler321_Spec_37_operator/1 -> xxeuler321_Spec_41_operator/2
  xxeuler321_Spec_44_operator/1 -> xxeuler321_Spec_45_operator/1
  xxeuler321_Spec_43_operator/1 -> xxeuler321_Spec_45_operator/2
  xxeuler321_Spec_45_operator/1 -> xxeuler321_Spec_46_operator/1
  xxeuler321_Spec_42_operator/1 -> xxeuler321_Spec_46_operator/2
  xxeuler321_Spec_4_rhs_2/1 -> xxeuler321_Spec_4_operator/2
  xxeuler321_Spec_49_operator/1 -> xxeuler321_Spec_50_operator/1
  xxeuler321_Spec_48_operator/1 -> xxeuler321_Spec_50_operator/2
  xxeuler321_Spec_50_operator/1 -> xxeuler321_Spec_51_operator/1
  xxeuler321_Spec_47_operator/1 -> xxeuler321_Spec_51_operator/2
  xxeuler321_Spec_54_operator/1 -> xxeuler321_Spec_55_operator/1
  xxeuler321_Spec_53_operator/1 -> xxeuler321_Spec_55_operator/2
  xxeuler321_Spec_55_operator/1 -> xxeuler321_Spec_56_operator/1
  xxeuler321_Spec_52_operator/1 -> xxeuler321_Spec_56_operator/2
  xxeuler321_Spec_5_rhs_2/1 -> xxeuler321_Spec_5_operator/2
  xxeuler321_Spec_59_operator/1 -> xxeuler321_Spec_60_operator/1
  xxeuler321_Spec_58_operator/1 -> xxeuler321_Spec_60_operator/2
  xxeuler321_Spec_60_operator/1 -> xxeuler321_Spec_61_operator/1
  xxeuler321_Spec_57_operator/1 -> xxeuler321_Spec_61_operator/2
  xxeuler321_Spec_63_cos_call/1 -> xxeuler321_Spec_64_operator/1
  xxeuler321_Spec_62_cos_call/1 -> xxeuler321_Spec_64_operator/2
  xxeuler321_Spec_66_sin_call/1 -> xxeuler321_Spec_67_operator/1
  xxeuler321_Spec_65_cos_call/1 -> xxeuler321_Spec_67_operator/2
  xxeuler321_Spec_68_sin_call/1 -> xxeuler321_Spec_69_operator/1
  r2xr1Transpose_operator/1 -> xxeuler321_Spec_6_operator/1
  xxeuler321_Spec_6_rhs_2/1 -> xxeuler321_Spec_6_operator/2
  xxeuler321_Spec_72_cos_call/1 -> xxeuler321_Spec_73_operator/1
  xxeuler321_Spec_71_sin_call/1 -> xxeuler321_Spec_73_operator/2
  xxeuler321_Spec_73_operator/1 -> xxeuler321_Spec_74_operator/1
  xxeuler321_Spec_70_sin_call/1 -> xxeuler321_Spec_74_operator/2
  xxeuler321_Spec_76_sin_call/1 -> xxeuler321_Spec_77_operator/1
  xxeuler321_Spec_77_operator/1 -> xxeuler321_Spec_78_operator/1
  xxeuler321_Spec_75_cos_call/1 -> xxeuler321_Spec_78_operator/2
  xxeuler321_Spec_78_operator/1 -> xxeuler321_Spec_79_operator/1
  xxeuler321_Spec_74_operator/1 -> xxeuler321_Spec_79_operator/2
  xxeuler321_Spec_7_rhs_2/1 -> xxeuler321_Spec_7_operator/2
  xxeuler321_Spec_82_sin_call/1 -> xxeuler321_Spec_83_operator/1
  xxeuler321_Spec_81_sin_call/1 -> xxeuler321_Spec_83_operator/2
  xxeuler321_Spec_83_operator/1 -> xxeuler321_Spec_84_operator/1
  xxeuler321_Spec_80_sin_call/1 -> xxeuler321_Spec_84_operator/2
  xxeuler321_Spec_86_cos_call/1 -> xxeuler321_Spec_87_operator/1
  xxeuler321_Spec_85_cos_call/1 -> xxeuler321_Spec_87_operator/2
  xxeuler321_Spec_87_operator/1 -> xxeuler321_Spec_88_operator/1
  xxeuler321_Spec_84_operator/1 -> xxeuler321_Spec_88_operator/2
  xxeuler321_Spec_8_rhs_2/1 -> xxeuler321_Spec_8_operator/2
  xxeuler321_Spec_90_cos_call/1 -> xxeuler321_Spec_91_operator/1
  xxeuler321_Spec_89_sin_call/1 -> xxeuler321_Spec_91_operator/2
  xxeuler321_Spec_94_cos_call/1 -> xxeuler321_Spec_95_operator/1
  xxeuler321_Spec_93_sin_call/1 -> xxeuler321_Spec_95_operator/2
  xxeuler321_Spec_95_operator/1 -> xxeuler321_Spec_96_operator/1
  xxeuler321_Spec_92_cos_call/1 -> xxeuler321_Spec_96_operator/2
  xxeuler321_Spec_98_sin_call/1 -> xxeuler321_Spec_99_operator/1
  xxeuler321_Spec_97_sin_call/1 -> xxeuler321_Spec_99_operator/2
  xxeuler321_Spec_9_rhs_2/1 -> xxeuler321_Spec_9_operator/2
  validator/1 -> valid/1
